simulink model "sfun_filter_model"  (R2013b)
settings: Solver=FixedStepDiscrete  StartTime=0.0  StopTime=30  FixedStep=0.01  RelTol=1e-3
settings Model: Creator=Administrator  LastModifiedBy=Administrator

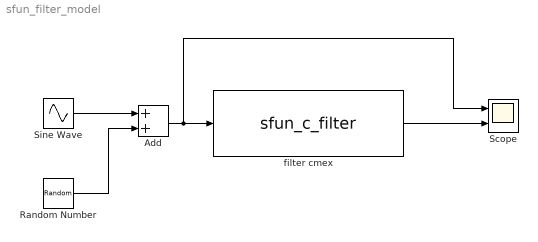
== system sfun_filter_model ==
  Add : Sum
  Random Number : RandomNumber
  Scope : Scope  NumInputPorts=2
      settings: YMin=-5~-5  YMax=5~5
  Sine Wave : Sin
  filter cmex : S-Function  FunctionName=sfun_c_filter  Parameters=g_coef  EnableBusSupport=off  mask(Custom by Hyo){g_coef=0.005}
      mask prompts: g_coef "Filter Coef"
      mask help:
      | This block simulates one order filter.
      | Its math model can be displayed as:
      | Y(t) = (U(t) – Y(t-1)) * Lc + Y(t – 1)
      mask Display: disp('Y(t) = (U(t) – Y(t-1)) * Lc + Y(t–1)');
  wires:
  Add/1 -> Scope/1, filter cmex/1
  Sine Wave/1 -> Add/1
  Random Number/1 -> Add/2
  filter cmex/1 -> Scope/2
